simulink model "PDPosition"  (R2021b)
settings: Solver=VariableStepAuto  StartTime=0.0  StopTime=1  RelTol=1e-3
libraries: aerolibutil x9, simulink x3, sharedutil x1, Contact_Forces_Lib x1, cstblocks x1, sharedtransform x1
settings Model: Creator=thinkpad  LastModifiedBy=thinkpad

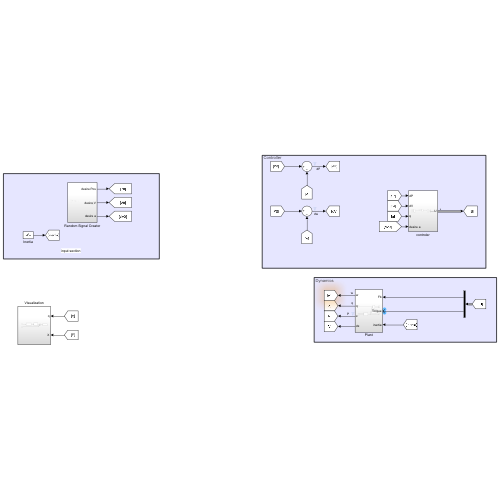
[thumbnail: Simulink's stored preview of the top-level diagram]
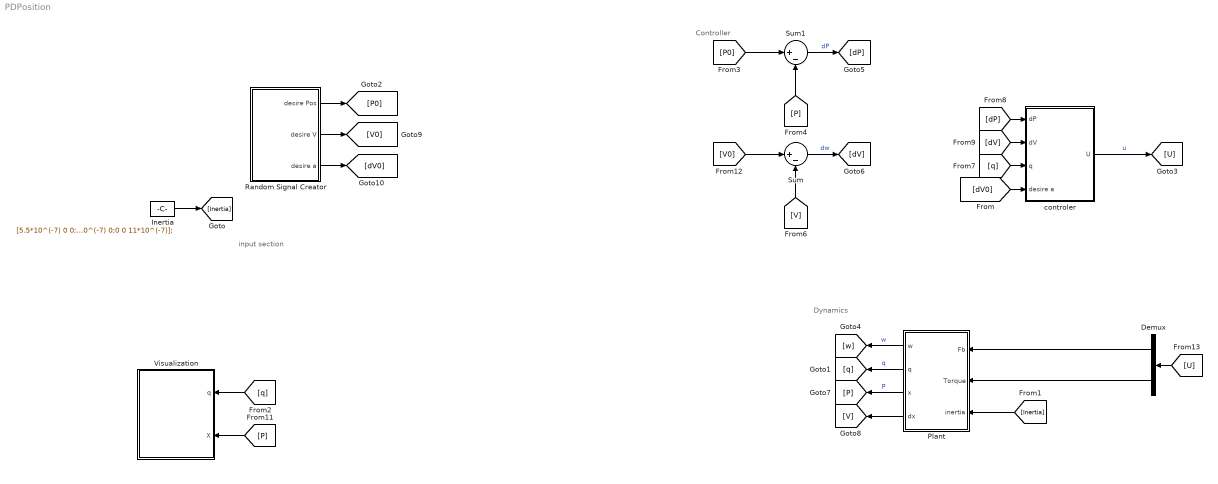
== system PDPosition ==
  note: input section
  note: Controller
  note: Dynamics
  Demux : Demux  Outputs=2
  Inertia : Constant  Value=[5.5*10^(-7) 0 0;0 5.5*10^(-7) 0;0 0 11*10^(-7)];
  Plant : Subsystem
  Random Signal Creator : Subsystem
  Sum : Sum  Inputs=|+-
  Sum1 : Sum  Inputs=|+-
  Visualization : Subsystem
  controler : Subsystem
  wires:
  Demux/2 -> Plant/2(Torque)
  [dV0] -> controler/4(desire a)
  Demux/1 -> Plant/1(Fb)
  [q] -> controler/3(q)
  [Inertia] -> Plant/3(inertia)
  Random Signal Creator/1(desire Pos) -> [P0]
  [q] -> Visualization/1(q)
  Plant/1(w) -> [w]  "w"
  [P] -> Visualization/2(X)
  Inertia/1 -> [Inertia]
  Plant/4(dx) -> [V]
  Plant/3(x) -> [P]  "P"
  Plant/2(q) -> [q]  "q"
  Sum/1 -> [dV]  "dw"
  [V] -> Sum/2
  Random Signal Creator/2(desire V) -> [V0]
  [V0] -> Sum/1
  [P] -> Sum1/2
  [P0] -> Sum1/1
  controler/1(U) -> [U]  "u"
  Sum1/1 -> [dP]  "dP"
  Random Signal Creator/3(desire a) -> [dV0]
  [U] -> Demux/1
  [dP] -> controler/1(dP)
  [dV] -> controler/2(dV)

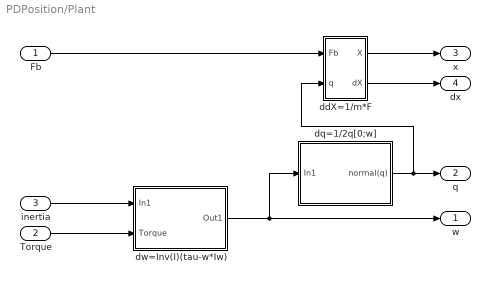
== system PDPosition/Plant ==
  Fb : Inport
  Torque : Inport  Port=2  PortDimensions=3
  inertia : Inport  Port=3
  ddX=1/m*F : Subsystem
  dq=1/2q[0;w] : Subsystem
  dw=Inv(I)(tau-w*Iw) : Subsystem
  w : Outport
  q : Outport  Port=2
  x : Outport  Port=3
  dx : Outport  Port=4
  wires:
  dw=Inv(I)(tau-w*Iw)/1(Out1) -> w/1, dq=1/2q[0;w]/1(In1)
  inertia/1 -> dw=Inv(I)(tau-w*Iw)/1(In1)
  Torque/1 -> dw=Inv(I)(tau-w*Iw)/2(Torque)
  dq=1/2q[0;w]/1(normal(q)) -> ddX=1/m*F/2(q), q/1
  Fb/1 -> ddX=1/m*F/1(Fb)
  ddX=1/m*F/1(X) -> x/1
  ddX=1/m*F/2(dX) -> dx/1

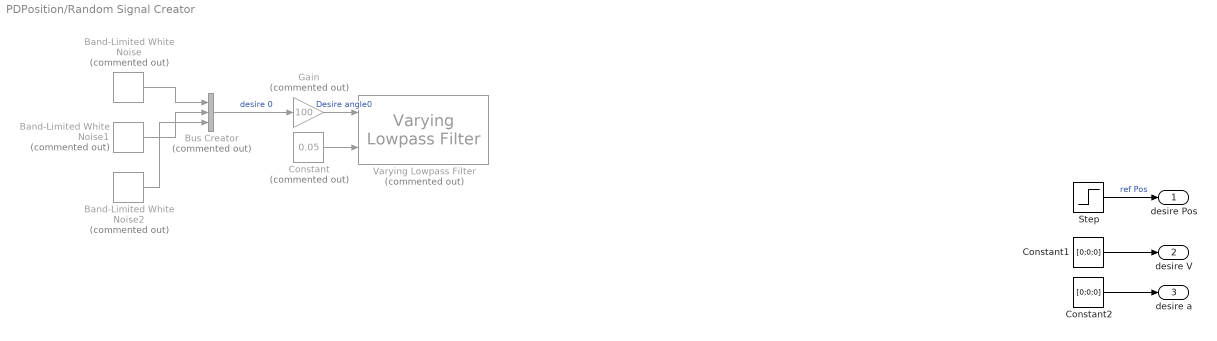
== system PDPosition/Random Signal Creator ==
  Band-Limited White Noise : simulink/Sources/Band-Limited White Noise  Commented=on  Cov=[0.005]  Ts=1e-3  seed=[23341]  VectorParams1D=off
  Band-Limited White Noise1 : simulink/Sources/Band-Limited White Noise  Commented=on  Cov=[0.005]  Ts=1e-3  seed=[23342]  VectorParams1D=off
  Band-Limited White Noise2 : simulink/Sources/Band-Limited White Noise  Commented=on  Cov=[0.005]  Ts=1e-3  seed=[23343]  VectorParams1D=off
  Bus Creator : BusCreator  Commented=on  Inputs=3
  Constant : Constant  Commented=on  Value=0.05
  Constant1 : Constant  Value=[0;0;0]
  Constant2 : Constant  Value=[0;0;0]
  Gain : Gain  Commented=on  Gain=100
  Step : Step  Time=0  Before=[0;0;0]  After=[1;1;1]  SampleTime=0
  Varying Lowpass Filter : cstblocks/Linear Parameter Varying/Varying Lowpass Filter  Commented=on  N=1
  desire Pos : Outport
  desire V : Outport  Port=2
  desire a : Outport  Port=3
  wires:
  Band-Limited White Noise1/1 -> Bus Creator/2
  Band-Limited White Noise2/1 -> Bus Creator/3
  Gain/1 -> Varying Lowpass Filter/1  "Desire angle0"
  Band-Limited White Noise/1 -> Bus Creator/1
  Bus Creator/1 -> Gain/1  "desire 0"
  Constant/1 -> Varying Lowpass Filter/2
  Constant2/1 -> desire a/1
  Constant1/1 -> desire V/1
  Step/1 -> desire Pos/1  "ref Pos"

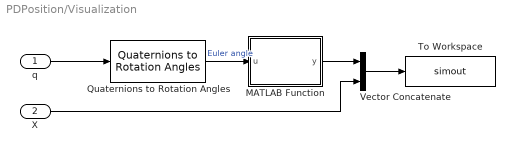
== system PDPosition/Visualization ==
  q : Inport
  X : Inport  Port=2
  MATLAB Function : MATLAB Function  TreatAsAtomicUnit=on
  Quaternions to Rotation Angles : sharedtransform/Quaternions to Rotation Angles  rotationOrder=ZYX  aMode=aMode
      settings: SourceProductBaseCode=AE,PW,DR,MT,UV,VE
  To Workspace : ToWorkspace  VariableName=simout  SampleTime=-1
      settings: Save2DSignal=2-D array (concatenate along first dimension)
  Vector Concatenate : Concatenate
  wires:
  q/1 -> Quaternions to Rotation Angles/1
  Quaternions to Rotation Angles/1 -> MATLAB Function/1(u)  "Euler angle"
  MATLAB Function/1(y) -> Vector Concatenate/1
  Vector Concatenate/1 -> To Workspace/1
  X/1 -> Vector Concatenate/2

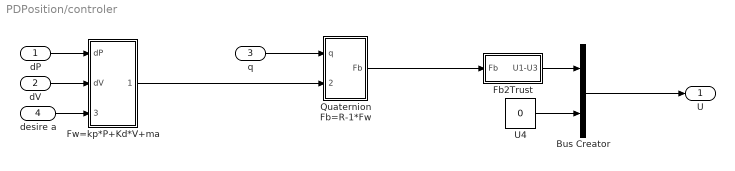
== system PDPosition/controler ==
  dP : Inport
  dV : Inport  Port=2  PortDimensions=3
  q : Inport  Port=3
  desire a : Inport  Port=4  PortDimensions=3
  Bus Creator : BusCreator  Inputs=2
  Fb2Trust : Subsystem
  Fw=kp*P+Kd*V+ma : Subsystem
  Quaternion Fb=R-1*Fw : Subsystem
  U4 : Constant  Value=0
  U : Outport
  wires:
  Bus Creator/1 -> U/1
  U4/1 -> Bus Creator/2
  Fb2Trust/1(U1-U3) -> Bus Creator/1
  dP/1 -> Fw=kp*P+Kd*V+ma/1(dP)
  dV/1 -> Fw=kp*P+Kd*V+ma/2(dV)
  desire a/1 -> Fw=kp*P+Kd*V+ma/3(desire a)
  q/1 -> Quaternion Fb=R-1*Fw/1(q)
  Fw=kp*P+Kd*V+ma/1(Out1) -> Quaternion Fb=R-1*Fw/2(Fb1)
  Quaternion Fb=R-1*Fw/1(Fb) -> Fb2Trust/1(Fb)

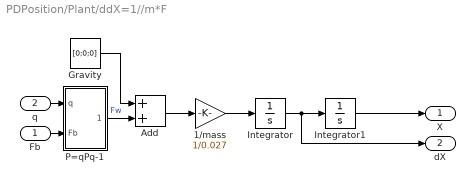
== system PDPosition/Plant/ddX=1//m*F ==
  Fb : Inport
  q : Inport  Port=2
  1/mass : Gain  Gain=1/0.027
  Add : Sum
  Gravity : Constant  Value=[0;0;0]
  Integrator : Integrator  InitialCondition=[0;0;0]
  Integrator1 : Integrator  InitialCondition=[0;0;0]
  P=qPq-1 : Subsystem
  X : Outport
  dX : Outport  Port=2
  wires:
  Integrator/1 -> dX/1, Integrator1/1
  Add/1 -> 1/mass/1
  Gravity/1 -> Add/1
  Integrator1/1 -> X/1
  q/1 -> P=qPq-1/1(q)
  Fb/1 -> P=qPq-1/2(Fb)
  P=qPq-1/1(Out1) -> Add/2  "Fw"
  1/mass/1 -> Integrator/1

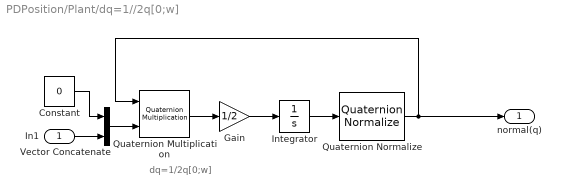
== system PDPosition/Plant/dq=1//2q[0;w] ==
  note: dq=1/2q[0;w]
  In1 : Inport
  Constant : Constant  Value=0
  Gain : Gain  Gain=1/2
  Integrator : Integrator  InitialCondition=[1;0;0;0]
  Quaternion Multiplication : aerolibutil/Quaternion Multiplication
  Quaternion Normalize : sharedutil/Quaternion Normalize  aMode=aMode
      settings: SourceProductBaseCode=AE,PW,DR,MT,UV,VE
  Vector Concatenate : Concatenate
  normal(q) : Outport
  wires:
  Quaternion Normalize/1 -> normal(q)/1, Quaternion Multiplication/1
  Integrator/1 -> Quaternion Normalize/1
  In1/1 -> Vector Concatenate/2
  Constant/1 -> Vector Concatenate/1
  Vector Concatenate/1 -> Quaternion Multiplication/2
  Quaternion Multiplication/1 -> Gain/1
  Gain/1 -> Integrator/1

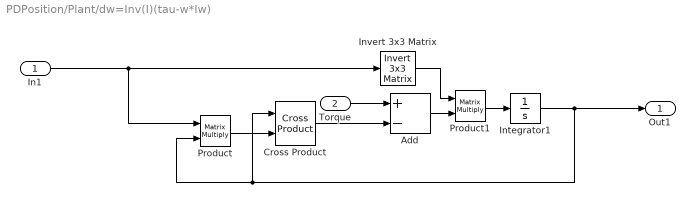
== system PDPosition/Plant/dw=Inv(I)(tau-w*Iw) ==
  In1 : Inport
  Torque : Inport  Port=2  PortDimensions=3
  Add : Sum  Inputs=+-
  Cross Product : Contact_Forces_Lib/Math/Cross Product  SystemSampleTime=-1  VariantActivationTime=update diagram  Latency=0  AutoFrameSizeCalculation=off
      settings: SourceProductName=Simscape Multibody Contact Forces Library
  Integrator1 : Integrator  InitialCondition=[0;0;0]
  Invert 3x3 Matrix : aerolibutil/Invert  3x3 Matrix
  Product : Product  Multiplication=Matrix(*)
  Product1 : Product  Multiplication=Matrix(*)
  Out1 : Outport
  wires:
  Product1/1 -> Integrator1/1
  Cross Product/1 -> Add/2
  Integrator1/1 -> Out1/1, Cross Product/1, Product/2
  Add/1 -> Product1/2
  In1/1 -> Invert 3x3 Matrix/1, Product/1
  Product/1 -> Cross Product/2
  Torque/1 -> Add/1
  Invert 3x3 Matrix/1 -> Product1/1

== system PDPosition/controler/Fb2Trust ==
  Fb : Inport
  Constant3 : Constant  Value=[0 0 1;0 1 0;1 0 0]
  Product : Product  Multiplication=Matrix(*)
  U1-U3 : Outport
  wires:
  Constant3/1 -> Product/1
  Product/1 -> U1-U3/1
  Fb/1 -> Product/2

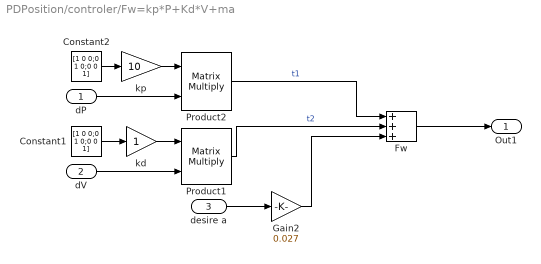
== system PDPosition/controler/Fw=kp*P+Kd*V+ma ==
  dP : Inport
  dV : Inport  Port=2  PortDimensions=3
  desire a : Inport  Port=3  PortDimensions=3
  Constant1 : Constant  Value=[1 0 0;0 1 0;0 0 1]
  Constant2 : Constant  Value=[1 0 0;0 1 0;0 0 1]
  Fw : Sum  Inputs=+++
  Gain2 : Gain  Gain=0.027
  Product1 : Product  Multiplication=Matrix(*)
  Product2 : Product  Multiplication=Matrix(*)
  kd : Gain
  kp : Gain  Gain=10
  Out1 : Outport
  wires:
  kd/1 -> Product1/1
  desire a/1 -> Gain2/1
  dP/1 -> Product2/2
  Product2/1 -> Fw/1  "t1"
  kp/1 -> Product2/1
  Constant1/1 -> kd/1
  dV/1 -> Product1/2
  Product1/1 -> Fw/2  "t2"
  Fw/1 -> Out1/1
  Constant2/1 -> kp/1
  Gain2/1 -> Fw/3

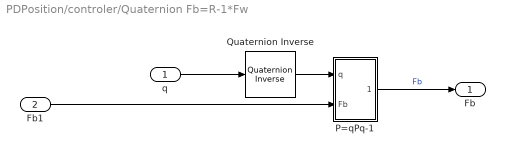
== system PDPosition/controler/Quaternion Fb=R-1*Fw ==
  q : Inport
  Fb1 : Inport  Port=2
  P=qPq-1 : Subsystem
  Quaternion Inverse : aerolibutil/Quaternion Inverse
  Fb : Outport
  wires:
  q/1 -> Quaternion Inverse/1
  P=qPq-1/1(Out1) -> Fb/1  "Fb"
  Quaternion Inverse/1 -> P=qPq-1/1(q)
  Fb1/1 -> P=qPq-1/2(Fb)

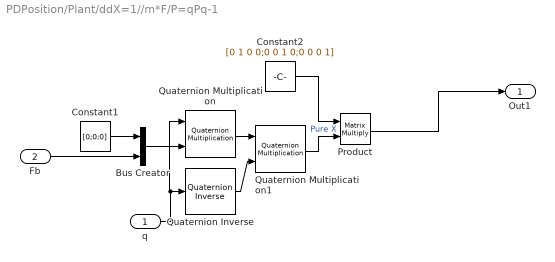
== system PDPosition/Plant/ddX=1//m*F/P=qPq-1 ==
  q : Inport
  Fb : Inport  Port=2
  Bus Creator : BusCreator  Inputs=2
  Constant1 : Constant  Value=[0;0;0]
  Constant2 : Constant  Value=[0 1 0 0;0 0 1 0;0 0 0 1]
  Product : Product  Multiplication=Matrix(*)
  Quaternion Inverse : aerolibutil/Quaternion Inverse
  Quaternion Multiplication : aerolibutil/Quaternion Multiplication
  Quaternion Multiplication1 : aerolibutil/Quaternion Multiplication
  Out1 : Outport
  wires:
  Quaternion Multiplication1/1 -> Product/2  "Pure X"
  q/1 -> Quaternion Multiplication/1, Quaternion Inverse/1
  Constant2/1 -> Product/1
  Bus Creator/1 -> Quaternion Multiplication/2
  Constant1/1 -> Bus Creator/1
  Quaternion Inverse/1 -> Quaternion Multiplication1/2
  Product/1 -> Out1/1
  Quaternion Multiplication/1 -> Quaternion Multiplication1/1
  Fb/1 -> Bus Creator/2

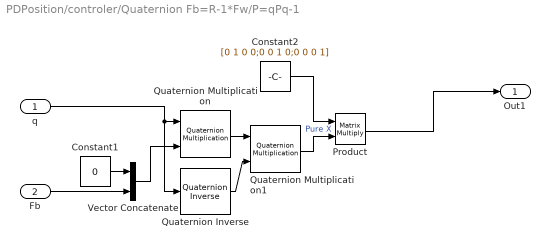
== system PDPosition/controler/Quaternion Fb=R-1*Fw/P=qPq-1 ==
  q : Inport
  Fb : Inport  Port=2
  Constant1 : Constant  Value=0
  Constant2 : Constant  Value=[0 1 0 0;0 0 1 0;0 0 0 1]
  Product : Product  Multiplication=Matrix(*)
  Quaternion Inverse : aerolibutil/Quaternion Inverse
  Quaternion Multiplication : aerolibutil/Quaternion Multiplication
  Quaternion Multiplication1 : aerolibutil/Quaternion Multiplication
  Vector Concatenate : Concatenate
  Out1 : Outport
  wires:
  Quaternion Multiplication1/1 -> Product/2  "Pure X"
  q/1 -> Quaternion Inverse/1, Quaternion Multiplication/1
  Constant2/1 -> Product/1
  Vector Concatenate/1 -> Quaternion Multiplication/2
  Constant1/1 -> Vector Concatenate/1
  Quaternion Inverse/1 -> Quaternion Multiplication1/2
  Product/1 -> Out1/1
  Quaternion Multiplication/1 -> Quaternion Multiplication1/1
  Fb/1 -> Vector Concatenate/2

== matlab function PDPosition/Visualization/MATLAB Function ==
  data: u input; y output
function y = fcn(u)
for i=1:3
    if u(i)> pi
        u(i)=u(i)-2*pi;
    end
end
y = u.';
